simulink model "2293_TP2_Parra"  (R2019b)
settings: Solver=ode4  StartTime=0.0  StopTime=10  FixedStep=10e-6  RelTol=1e-3
libraries: cstblocks x2
settings Model: Creator=mpier  LastModifiedBy=rochi

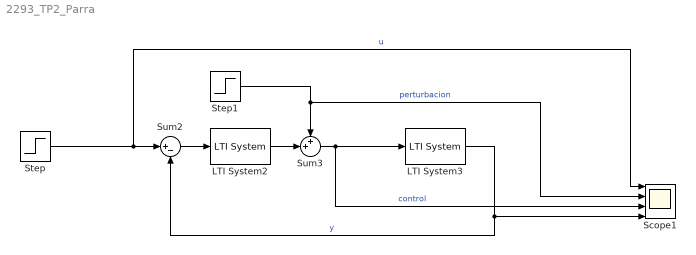
== system 2293_TP2_Parra ==
  LTI System2 : cstblocks/LTI System  sys=c_disc  IC=[]
  LTI System3 : cstblocks/LTI System  sys=planta_disc  IC=[]
  Scope1 : Scope  NumInputPorts=4
  Step : Step  SampleTime=0
  Step1 : Step  Time=5  After=10  SampleTime=0
  Sum2 : Sum  Inputs=|+-
  Sum3 : Sum  Inputs=++|
  wires:
  Step/1 -> Scope1/1, Sum2/1  "u"
  Step1/1 -> Sum3/1, Scope1/2  "perturbacion"
  Sum2/1 -> LTI System2/1
  LTI System3/1 -> Sum2/2, Scope1/4  "y"
  LTI System2/1 -> Sum3/2
  Sum3/1 -> Scope1/3, LTI System3/1  "control"
